simulink model "sdslip1r"  (Simulink 5.0)
settings: Solver=ode45  StartTime=0.0  StopTime=tsim  RelTol=1e-5
values from neighbouring files (symbols this model uses):
  dstepr = u0/R    (= 0.07)    [tslip1.m]
  f2 = inv(dcg2)    [tslip1.m]
  k2 = lqrd(a2,b2,eye(2),1,Ts)    [tslip1.m]
  k3 = lqrd(a3,b3,eye(3),diag([1 .01/1000]),Ts)    [tslip1.m]
  T0 = 44*(u0/10)^2;Vi(1)=u0    [tslip1.m]
  Ts = 0.1    [start.m]    (also in tslip1.m = 0.05)
  tstepdd = 5    [tslip1.m]
  u0 = x(13)    [smis30.m]    (also in tslip1.m = 3.5)
  Vi = XU0(1:7)    [tslip1.m]
settings Model: LastModifiedBy=jra

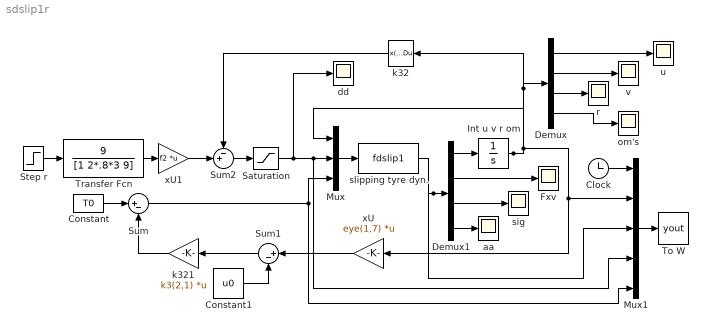
== system sdslip1r ==
  Clock : Clock
      settings: Decimation=10
  Constant : Constant  Value=T0
  Constant1 : Constant  Value=u0
  Demux : Demux  Outputs=[1 1 1 4]
  Demux1 : Demux  Outputs=[7 4 4 4]
  Fxv : Scope
      settings: YMin=-7.5  YMax=20  SaveName=ScopeData5
  Int u v r om : Integrator  InitialCondition=Vi
  Mux : Mux  Inputs=[7 1 1]
  Mux1 : Mux  Inputs=[1 7 19 1 1]
  Saturation : Saturate  UpperLimit=0.49  LowerLimit=-0.49
  Step r : Step  Time=tstepdd  After=dstepr  SampleTime=0
  Sum : Sum  Inputs=|+-  SaturateOnIntegerOverflow=on
  Sum1 : Sum  Orientation=left  Inputs=|+-  SaturateOnIntegerOverflow=on
  Sum2 : Sum  Inputs=-+|  SaturateOnIntegerOverflow=on
  To W : ToWorkspace  VariableName=yout  SampleTime=-1  SaveFormat=Array
  Transfer Fcn : TransferFcn  Numerator=[9]  Denominator=[1 2*.8*3 9]
  aa : Scope
      settings: YMin=-0.0013  YMax=-0.0003  SaveName=ScopeData7
  dd : Scope
      settings: YMin=-0.5  YMax=0.5  SaveName=ScopeData3
  k32 : DiscreteStateSpace  Orientation=left  A=[]  B=[]  C=[]  D=k2*[0 1 0;0 0 1]*eye(3,7)  SampleTime=Ts
  k321 : Gain  Orientation=left  Gain=k3(2,1)  Multiplication=Matrix(K*u)  SaturateOnIntegerOverflow=on
  om's : Scope
      settings: YMin=19.6  YMax=20.4  SaveName=ScopeData4
  r : Scope
      settings: YMin=0  YMax=0.15
  sig : Scope
      settings: YMin=-0.001  YMax=0.00075  SaveName=ScopeData6
  slipping tyre dyn. : MATLABFcn  MATLABFcn=fdslip1  OutputDimensions=3+4+3*4
  u : Scope
      settings: YMin=0  YMax=50  SaveName=ScopeData2
  v : Scope
      settings: YMin=0  YMax=0.2
  xU : Gain  Orientation=left  Gain=eye(1,7)  Multiplication=Matrix(K*u)  SaturateOnIntegerOverflow=on
  xU1 : Gain  Gain=f2  Multiplication=Matrix(K*u)  SaturateOnIntegerOverflow=on
  wires:
  Mux/1 -> slipping tyre dyn./1
  slipping tyre dyn./1 -> Demux1/1, Mux1/3
  Int u v r om/1 -> Mux/1, Mux1/2, xU/1, Demux/1, k32/1
  Demux/1 -> u/1
  Demux/2 -> v/1
  Saturation/1 -> dd/1, Mux/2, Mux1/4
  Demux/3 -> r/1
  Demux/4 -> om's/1
  Step r/1 -> Transfer Fcn/1
  Demux1/1 -> Int u v r om/1
  Demux1/2 -> Fxv/1
  Demux1/3 -> sig/1
  Demux1/4 -> aa/1
  Mux1/1 -> To W/1
  Clock/1 -> Mux1/1
  Sum1/1 -> k321/1
  Constant1/1 -> Sum1/2
  xU/1 -> Sum1/1
  Constant/1 -> Sum/1
  Sum/1 -> Mux/3, Mux1/5
  k321/1 -> Sum/2
  Sum2/1 -> Saturation/1
  k32/1 -> Sum2/1
  xU1/1 -> Sum2/2
  Transfer Fcn/1 -> xU1/1
